simulink model "gm_sampleModel1959_2_sub"  (R2023a)
settings: Solver=VariableStepAuto  StartTime=0.0  StopTime=10.0  RelTol=1e-3
libraries: simulink x1
settings Model: Creator=user1  LastModifiedBy=user1
settings OptimizationCC: BlockReduction=off  ConditionallyExecuteInputs=off
settings DebuggingCC: InheritedTsInSrcMsg=none

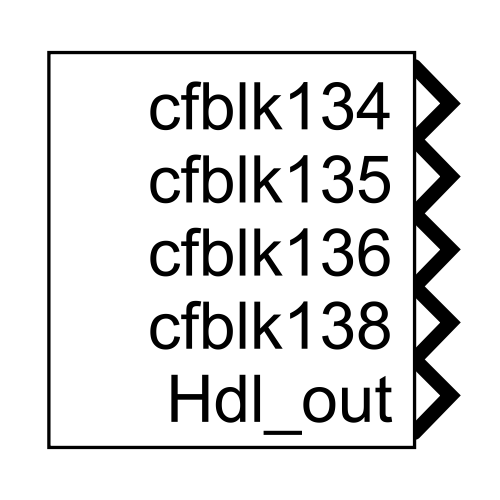
[thumbnail: Simulink's stored preview of the top-level diagram]
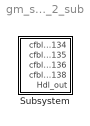
== system gm_sampleModel1959_2_sub ==
  Subsystem : Subsystem

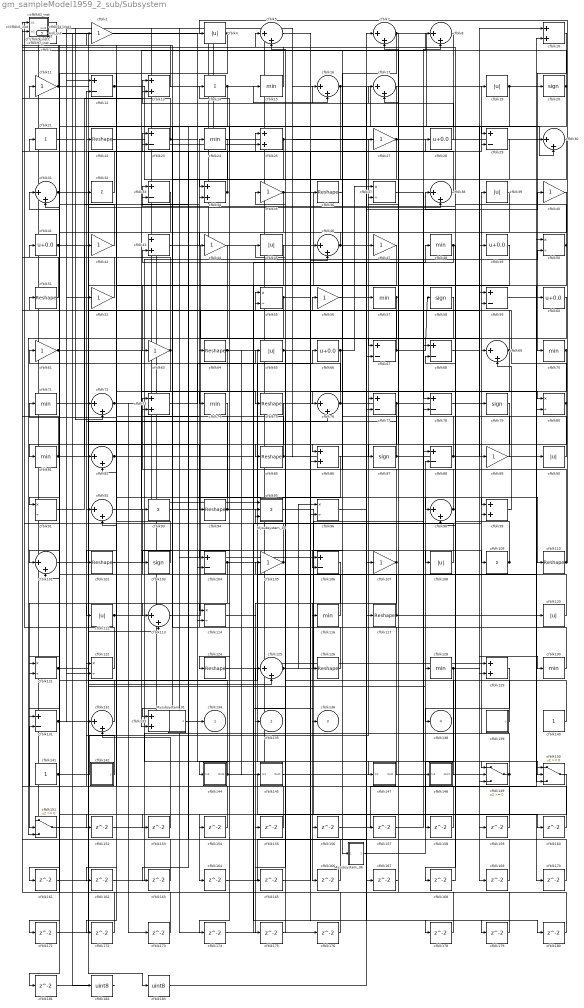
== system gm_sampleModel1959_2_sub/Subsystem ==
  Mysubsystem_15 : Subsystem
  Mysubsystem_31 : Subsystem
  Mysubsystem_36 : Subsystem
  cfblk1 : simulink/Logic and Bit Operations/Bit Clear  iBit=0
      settings: LibrarySourceBlock=|
      | hdlsllib/Logic and Bit
      | Operations/Bit Clear
  cfblk{10,13,25,34,43,73,86,99,129,133} (10 alike) : Sum  OutDataTypeStr=uint8
  cfblk100_inst : Subsystem
  cfblk{5,7..8,16..17,30..31,38,46,69,72,76,82,92,98,101,113,125,132} (19 alike) : Sum  Inputs=|++  OutDataTypeStr=uint8
  cfblk{22,36,51,64,75,85,94,102,110,117,124,126} (12 alike) : Reshape
  cfblk{20,58,79,87,103} (5 alike) : Signum
  cfblk{12,23,29,33,59,67..68,77..78,88,104,106,131} (13 alike) : Sum  Inputs=+-  OutDataTypeStr=uint8
  cfblk{2,11,27,35,40,42,44,47,52,56,61,63,89,105,107} (15 alike) : Gain  OutDataTypeStr=uint8
  cfblk{4,19,39,45,65,90,108,112,120} (9 alike) : Abs  OutDataTypeStr=uint8  SaturateOnIntegerOverflow=off
  cfblk{14,21,32,93,95,109} (6 alike) : Sum  Inputs=+  OutDataTypeStr=uint8
  cfblk111_inst : Subsystem
  cfblk{37,50,55,80,91,96,114,121..122} (9 alike) : Product  Inputs=*/  OutDataTypeStr=uint8  RndMeth=Zero  SaturateOnIntegerOverflow=on
  cfblk115_inst : Subsystem
  cfblk{15,24,48,57,70..71,74,81,116,128,130} (11 alike) : MinMax  OutDataTypeStr=uint8
  cfblk119_inst : Subsystem
  cfblk127_inst : Subsystem
  cfblk139 : Subsystem  mask(Counter Free-Running){NumBits=double(16), tsamp=double(-1)}
      mask prompts: NumBits "Simulink:masks:NumberOfBits_MP"; tsamp "Simulink:masks:SampleTime_MP"
      mask help: Simulink:masks:CounterFreeRunning_MD
  cfblk140 : Constant  OutDataTypeStr=uint8  SampleTime=-1
  cfblk141 : Constant  OutDataTypeStr=uint8  SampleTime=-1
  cfblk142 : Subsystem  mask(Counter Limited){uplimit=double(7), tsamp=double(-1)}
      mask prompts: uplimit "Simulink:masks:UpperLimit_MP"; tsamp "Simulink:masks:SampleTime_MP"
      mask help: Simulink:masks:CounterLimited_MD
      mask init:
      | nbits = double(8);
      | tsamp = double(-1);
      | uplimit = double(7);
  cfblk144 : Subsystem
  cfblk145 : Subsystem
  cfblk147 : Subsystem
  cfblk148 : Subsystem
  cfblk149 : Switch  OutDataTypeStr=uint8  SaturateOnIntegerOverflow=off  InputSameDT=off
  cfblk150 : Switch  OutDataTypeStr=uint8  SaturateOnIntegerOverflow=off  InputSameDT=off
  cfblk151 : Switch  OutDataTypeStr=uint8  SaturateOnIntegerOverflow=off  InputSameDT=off
  cfblk{152..176,178..181} (29 alike) : Delay  SampleTime=1
  cfblk182 : DataTypeConversion  OutDataTypeStr=uint8  SaturateOnIntegerOverflow=off  RndMeth=Floor
  cfblk183 : DataTypeConversion  OutDataTypeStr=uint8  SaturateOnIntegerOverflow=off  RndMeth=Floor
  cfblk18_inst : Subsystem
  cfblk26_inst : Subsystem
  cfblk{28,41,49,60,66} (5 alike) : Bias  Bias=0.0  SaturateOnIntegerOverflow=off
  cfblk3_inst : Subsystem
  cfblk53_inst : Subsystem
  cfblk54_inst : Subsystem
  cfblk62_inst : Subsystem
  cfblk6_inst : Subsystem
  cfblk97_inst : Subsystem
  cfblk9_inst : Subsystem
  cfblk134 : Outport  OutDataTypeStr=uint8  SampleTime=1  VectorParamsAs1DForOutWhenUnconnected=off
  cfblk135 : Outport  Port=2  OutDataTypeStr=uint8  SampleTime=1  VectorParamsAs1DForOutWhenUnconnected=off
  cfblk136 : Outport  Port=3  OutDataTypeStr=uint8  SampleTime=1  VectorParamsAs1DForOutWhenUnconnected=off
  cfblk138 : Outport  Port=4  OutDataTypeStr=uint8  SampleTime=1  VectorParamsAs1DForOutWhenUnconnected=off
  Hdl_out : Outport  Port=5  OutDataTypeStr=uint8  SampleTime=1
  wires:
  Mysubsystem_15/1(Out1) -> cfblk160/1
  Mysubsystem_31/1(cfblk134) -> cfblk134/1
  Mysubsystem_36/1(Out1) -> cfblk88/2
  cfblk1/1 -> cfblk183/1
  cfblk10/1 -> cfblk70/1
  cfblk100_inst/1(out1) -> cfblk12/1
  cfblk101/1 -> cfblk125/2
  cfblk102/1 -> cfblk50/2
  cfblk103/1 -> cfblk71/1
  cfblk104/1 -> cfblk151/2, cfblk149/1
  cfblk105/1 -> cfblk66/1, cfblk53_inst/1(in1)
  cfblk106/1 -> cfblk175/1
  cfblk107/1 -> cfblk73/1, cfblk166/1, Mysubsystem_15/2(In2)
  cfblk108/1 -> Mysubsystem_15/3(In3)
  cfblk109/1 -> cfblk33/1, cfblk100_inst/1(in1)
  cfblk11/1 -> cfblk62_inst/1(in1), cfblk38/2
  cfblk110/1 -> cfblk4/1, cfblk17/2
  cfblk111_inst/1(out1) -> cfblk15/1
  cfblk112/1 -> cfblk147/1(In1), cfblk24/1
  cfblk113/1 -> cfblk56/1
  cfblk114/1 -> cfblk155/1
  cfblk115_inst/1(out1) -> cfblk9_inst/1(in1), cfblk72/2, cfblk149/2
  cfblk116/1 -> cfblk12/2
  cfblk117/1 -> cfblk120/1, cfblk61/1
  cfblk119_inst/1(out1) -> cfblk176/1
  cfblk12/1 -> cfblk86/2, cfblk96/2
  cfblk120/1 -> cfblk93/1
  cfblk121/1 -> cfblk76/2, cfblk55/1
  cfblk122/1 -> cfblk18_inst/2(in2)
  cfblk124/1 -> cfblk27/1
  cfblk125/1 -> cfblk88/1, cfblk96/1
  cfblk126/1 -> cfblk2/1
  cfblk127_inst/1(out1) -> cfblk47/1
  cfblk128/1 -> cfblk159/1, cfblk158/1
  cfblk129/1 -> cfblk138/1
  cfblk13/1 -> cfblk115_inst/1(in1)
  cfblk130/1 -> cfblk45/1
  cfblk131/1 -> cfblk73/2, cfblk113/2, cfblk128/1
  cfblk132/1 -> cfblk31/2
  cfblk133/1 -> cfblk43/1
  cfblk139/1(y) -> cfblk25/1
  cfblk14/1 -> cfblk16/2, cfblk133/1
  cfblk140/1 -> cfblk38/1
  cfblk141/1 -> cfblk77/1, cfblk101/2
  cfblk142/1(y) -> cfblk22/1
  cfblk144/1(Out1) -> cfblk41/1, cfblk170/1
  cfblk145/1(Out1) -> cfblk179/1
  cfblk147/1(Out1) -> cfblk64/1
  cfblk148/1(Out1) -> cfblk105/1
  cfblk149/1 -> cfblk39/1, cfblk161/1
  cfblk15/1 -> cfblk5/1
  cfblk150/1 -> cfblk164/1
  cfblk151/1 -> cfblk19/1
  cfblk152/1 -> cfblk69/1
  cfblk153/1 -> cfblk132/2
  cfblk154/1 -> cfblk122/1
  cfblk155/1 -> cfblk6_inst/2(in2)
  cfblk156/1 -> cfblk50/1
  cfblk157/1 -> cfblk78/2
  cfblk158/1 -> cfblk92/1
  cfblk159/1 -> cfblk33/2
  cfblk16/1 -> cfblk149/3, cfblk113/1, cfblk167/1
  cfblk160/1 -> cfblk131/2
  cfblk161/1 -> cfblk10/2
  cfblk162/1 -> cfblk8/2
  cfblk163/1 -> cfblk54_inst/2(in2)
  cfblk164/1 -> cfblk67/2
  cfblk165/1 -> cfblk46/2
  cfblk166/1 -> cfblk23/1
  cfblk167/1 -> cfblk37/2
  cfblk168/1 -> cfblk68/2
  cfblk169/1 -> cfblk26_inst/2(in2)
  cfblk17/1 -> cfblk154/1
  cfblk170/1 -> cfblk5/2
  cfblk171/1 -> cfblk125/1
  cfblk172/1 -> cfblk18_inst/1(in1)
  cfblk173/1 -> cfblk111_inst/2(in2)
  cfblk174/1 -> cfblk99/2
  cfblk175/1 -> cfblk55/2
  cfblk176/1 -> cfblk31/1
  cfblk178/1 -> cfblk7/2
  cfblk179/1 -> cfblk97_inst/2(in2)
  cfblk18_inst/1(out1) -> cfblk25/2
  cfblk180/1 -> cfblk3_inst/1(in1)
  cfblk181/1 -> cfblk182/1
  cfblk182/1 -> cfblk1/1
  cfblk183/1 -> cfblk7/1
  cfblk19/1 -> cfblk163/1, cfblk162/1
  cfblk2/1 -> cfblk99/1
  cfblk20/1 -> cfblk62_inst/2(in2), cfblk156/1
  cfblk21/1 -> cfblk29/1
  cfblk22/1 -> cfblk57/1
  cfblk23/1 -> cfblk115_inst/2(in2), cfblk148/1(In1)
  cfblk24/1 -> cfblk103/1
  cfblk25/1 -> cfblk23/2, cfblk153/1
  cfblk26_inst/1(out1) -> cfblk52/1
  cfblk27/1 -> cfblk174/1, Hdl_out/1
  cfblk28/1 -> cfblk13/1
  cfblk29/1 -> cfblk144/1(In1)
  cfblk3_inst/1(out1) -> cfblk90/1, Mysubsystem_15/1(In1)
  cfblk30/1 -> cfblk34/1
  cfblk31/1 -> cfblk63/1, cfblk32/1
  cfblk32/1 -> cfblk26_inst/1(in1)
  cfblk33/1 -> cfblk131/1
  cfblk34/1 -> cfblk119_inst/2(in2), cfblk119_inst/1(in1)
  cfblk35/1 -> cfblk80/2, cfblk121/2, cfblk81/1
  cfblk36/1 -> cfblk116/1
  cfblk37/1 -> cfblk78/1
  cfblk38/1 -> cfblk14/1
  cfblk39/1 -> cfblk114/1
  cfblk4/1 -> cfblk172/1, cfblk121/1
  cfblk40/1 -> cfblk77/2
  cfblk41/1 -> cfblk82/1, cfblk169/1
  cfblk42/1 -> cfblk111_inst/1(in1)
  cfblk43/1 -> cfblk89/1
  cfblk44/1 -> cfblk171/1
  cfblk45/1 -> cfblk92/2
  cfblk46/1 -> cfblk117/1, cfblk44/1
  cfblk47/1 -> cfblk95/1
  cfblk48/1 -> cfblk98/2, cfblk43/2
  cfblk49/1 -> cfblk67/1
  cfblk5/1 -> cfblk126/1
  cfblk50/1 -> cfblk60/1, cfblk53_inst/2(in2)
  cfblk51/1 -> cfblk100_inst/2(in2)
  cfblk52/1 -> cfblk42/1
  cfblk53_inst/1(out1) -> cfblk20/1, cfblk151/1
  cfblk54_inst/1(out1) -> cfblk97_inst/1(in1), cfblk79/1
  cfblk55/1 -> cfblk28/1, cfblk104/1
  cfblk56/1 -> cfblk107/1
  cfblk57/1 -> cfblk151/3, cfblk91/1
  cfblk58/1 -> cfblk74/1
  cfblk59/1 -> cfblk150/3
  cfblk6_inst/1(out1) -> cfblk132/1
  cfblk60/1 -> cfblk86/1
  cfblk61/1 -> cfblk29/2, cfblk109/1
  cfblk62_inst/1(out1) -> cfblk46/1, cfblk129/1
  cfblk63/1 -> cfblk82/2, cfblk127_inst/2(in2), cfblk127_inst/1(in1)
  cfblk64/1 -> cfblk110/1, cfblk102/1, cfblk145/1(In1)
  cfblk65/1 -> cfblk108/1, cfblk80/1, cfblk165/1
  cfblk66/1 -> cfblk133/2, cfblk106/2, cfblk37/1
  cfblk67/1 -> cfblk58/1, cfblk35/1
  cfblk68/1 -> cfblk49/1
  cfblk69/1 -> cfblk3_inst/2(in2), cfblk135/1
  cfblk7/1 -> cfblk87/1, cfblk76/1, cfblk30/2
  cfblk70/1 -> cfblk129/2, cfblk112/1
  cfblk71/1 -> cfblk94/1
  cfblk72/1 -> cfblk75/1, cfblk173/1
  cfblk73/1 -> cfblk65/1
  cfblk74/1 -> cfblk152/1
  cfblk75/1 -> cfblk124/1
  cfblk76/1 -> cfblk40/1, cfblk11/1, Mysubsystem_36/1(In1)
  cfblk77/1 -> cfblk85/1, cfblk150/2
  cfblk78/1 -> cfblk130/1
  cfblk79/1 -> cfblk181/1
  cfblk8/1 -> cfblk101/1
  cfblk80/1 -> cfblk59/2, cfblk104/2
  cfblk81/1 -> cfblk54_inst/1(in1), cfblk34/2
  cfblk82/1 -> cfblk136/1, cfblk48/1
  cfblk85/1 -> cfblk98/1, cfblk178/1, cfblk21/1
  cfblk86/1 -> cfblk114/2
  cfblk87/1 -> cfblk72/1, cfblk6_inst/1(in1)
  cfblk88/1 -> cfblk17/1, cfblk10/1
  cfblk89/1 -> cfblk51/1
  cfblk9_inst/1(out1) -> cfblk30/1, cfblk106/1
  cfblk90/1 -> cfblk68/1
  cfblk91/1 -> cfblk13/2
  cfblk92/1 -> cfblk8/1
  cfblk93/1 -> cfblk150/1
  cfblk94/1 -> cfblk9_inst/2(in2), cfblk59/1, cfblk180/1
  cfblk95/1 -> cfblk36/1
  cfblk96/1 -> cfblk157/1
  cfblk97_inst/1(out1) -> cfblk91/2, cfblk122/2
  cfblk98/1 -> cfblk16/1, cfblk168/1
  cfblk99/1 -> cfblk69/2

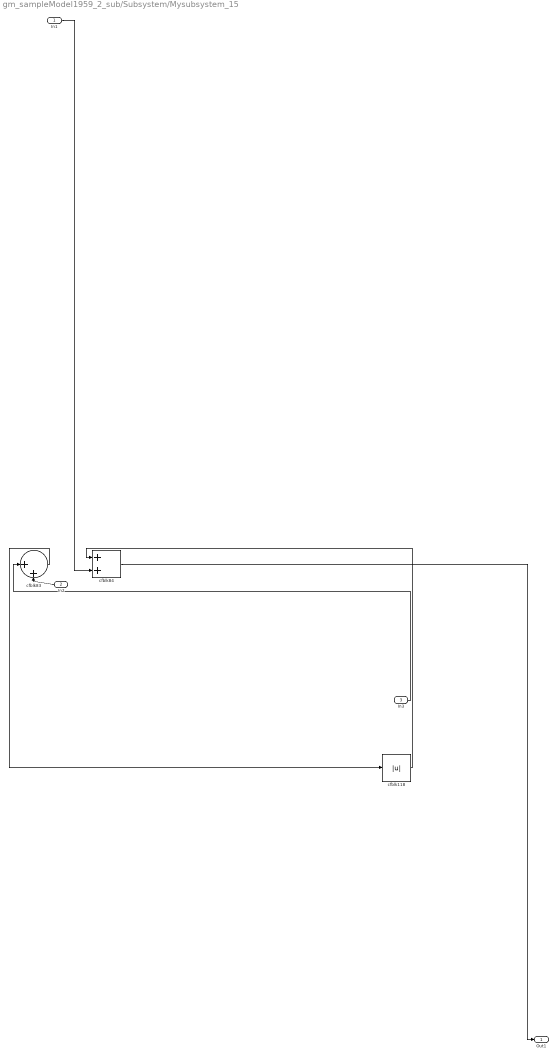
== system gm_sampleModel1959_2_sub/Subsystem/Mysubsystem_15 ==
  In1 : Inport  OutDataTypeStr=uint8  PortDimensions=1  SampleTime=1
  In2 : Inport  Port=2  OutDataTypeStr=uint8  PortDimensions=1  SampleTime=1
  In3 : Inport  Port=3  OutDataTypeStr=uint8  PortDimensions=1  SampleTime=1
  cfblk118 : Abs  SaturateOnIntegerOverflow=off
  cfblk83 : Sum  Inputs=|++
  cfblk84 : Sum
  Out1 : Outport  SampleTime=1
  wires:
  In1/1 -> cfblk84/2
  In2/1 -> cfblk83/2
  In3/1 -> cfblk83/1
  cfblk118/1 -> cfblk84/1
  cfblk83/1 -> cfblk118/1
  cfblk84/1 -> Out1/1

== system gm_sampleModel1959_2_sub/Subsystem/Mysubsystem_31 ==
  cfblk123 : Abs  SaturateOnIntegerOverflow=off
  cfblk143 : Subsystem  mask(Counter Limited){uplimit=double(7), tsamp=double(-1)}
      mask prompts: uplimit "Simulink:masks:UpperLimit_MP"; tsamp "Simulink:masks:SampleTime_MP"
      mask help: Simulink:masks:CounterLimited_MD
      mask init:
      | nbits = double(8);
      | tsamp = double(-1);
      | uplimit = double(7);
  cfblk134 : Outport  SampleTime=1  VectorParamsAs1DForOutWhenUnconnected=off
  wires:
  cfblk123/1 -> cfblk134/1
  cfblk143/1(y) -> cfblk123/1

== system gm_sampleModel1959_2_sub/Subsystem/Mysubsystem_36 ==
  In1 : Inport  OutDataTypeStr=uint8  PortDimensions=1  SampleTime=1
  cfblk146 : Subsystem
  cfblk177 : Delay  SampleTime=1
  Out1 : Outport  SampleTime=1
  wires:
  In1/1 -> cfblk146/1(In1)
  cfblk146/1(Out1) -> cfblk177/1
  cfblk177/1 -> Out1/1

== system gm_sampleModel1959_2_sub/Subsystem/cfblk100_inst ==
  in1 : Inport  OutDataTypeStr=uint8  SampleTime=1
  in2 : Inport  Port=2  OutDataTypeStr=uint8  SampleTime=1
  mul_cfblk100_dotp_mulcomp : Product  Inputs=**  OutDataTypeStr=uint8  SampleTime=1
  out1 : Outport  OutDataTypeStr=uint8  SampleTime=1
  wires:
  in1/1 -> mul_cfblk100_dotp_mulcomp/1
  in2/1 -> mul_cfblk100_dotp_mulcomp/2
  mul_cfblk100_dotp_mulcomp/1 -> out1/1

== system gm_sampleModel1959_2_sub/Subsystem/cfblk111_inst ==
  in1 : Inport  OutDataTypeStr=uint8  SampleTime=1
  in2 : Inport  Port=2  OutDataTypeStr=uint8  SampleTime=1
  mul_cfblk111_dotp_mulcomp : Product  Inputs=**  OutDataTypeStr=uint8  SampleTime=1
  out1 : Outport  OutDataTypeStr=uint8  SampleTime=1
  wires:
  in1/1 -> mul_cfblk111_dotp_mulcomp/1
  in2/1 -> mul_cfblk111_dotp_mulcomp/2
  mul_cfblk111_dotp_mulcomp/1 -> out1/1

== system gm_sampleModel1959_2_sub/Subsystem/cfblk115_inst ==
  in1 : Inport  OutDataTypeStr=uint8  SampleTime=1
  in2 : Inport  Port=2  OutDataTypeStr=uint8  SampleTime=1
  mul_cfblk115_dotp_mulcomp : Product  Inputs=**  OutDataTypeStr=uint8  SampleTime=1
  out1 : Outport  OutDataTypeStr=uint8  SampleTime=1
  wires:
  in1/1 -> mul_cfblk115_dotp_mulcomp/1
  in2/1 -> mul_cfblk115_dotp_mulcomp/2
  mul_cfblk115_dotp_mulcomp/1 -> out1/1

== system gm_sampleModel1959_2_sub/Subsystem/cfblk119_inst ==
  in1 : Inport  OutDataTypeStr=uint8  SampleTime=1
  in2 : Inport  Port=2  OutDataTypeStr=uint8  SampleTime=1
  mul_cfblk119_dotp_mulcomp : Product  Inputs=**  OutDataTypeStr=uint8  SampleTime=1
  out1 : Outport  OutDataTypeStr=uint8  SampleTime=1
  wires:
  in1/1 -> mul_cfblk119_dotp_mulcomp/1
  in2/1 -> mul_cfblk119_dotp_mulcomp/2
  mul_cfblk119_dotp_mulcomp/1 -> out1/1

== system gm_sampleModel1959_2_sub/Subsystem/cfblk127_inst ==
  in1 : Inport  OutDataTypeStr=uint8  SampleTime=1
  in2 : Inport  Port=2  OutDataTypeStr=uint8  SampleTime=1
  mul_cfblk127_dotp_mulcomp : Product  Inputs=**  OutDataTypeStr=uint8  SampleTime=1
  out1 : Outport  OutDataTypeStr=uint8  SampleTime=1
  wires:
  in1/1 -> mul_cfblk127_dotp_mulcomp/1
  in2/1 -> mul_cfblk127_dotp_mulcomp/2
  mul_cfblk127_dotp_mulcomp/1 -> out1/1

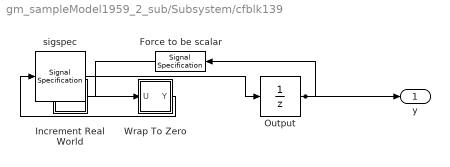
== system gm_sampleModel1959_2_sub/Subsystem/cfblk139 ==
  Force to be scalar : SignalSpecification  DisableCoverage=on  Dimensions=1
  Increment Real World : Subsystem  mask(Real World Value Increment){}
      mask help: Simulink:masks:RealWorldValueIncrement_MD
      mask Display: disp('V++')
  Output : UnitDelay  InitialCondition=0.0  SampleTime=tsamp  HasFrameUpgradeWarning=on
  Wrap To Zero : Subsystem  mask(Wrap To Zero){Threshold=double(65535)}
      mask prompts: Threshold "Simulink:masks:Threshold_MP"
      mask help: Simulink:masks:WrapToZero_MD
  sigspec : SignalSpecification  OutDataTypeStr=uint16  Dimensions=1
  y : Outport  SampleTime=1
  wires:
  Force to be scalar/1 -> Increment Real World/1(u)
  Increment Real World/1(y) -> Wrap To Zero/1(U)
  Output/1 -> Force to be scalar/1, y/1
  Wrap To Zero/1(Y) -> sigspec/1
  sigspec/1 -> Output/1

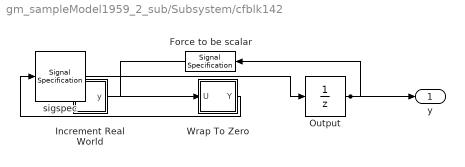
== system gm_sampleModel1959_2_sub/Subsystem/cfblk142 ==
  Force to be scalar : SignalSpecification  DisableCoverage=on  Dimensions=1
  Increment Real World : Subsystem  mask(Real World Value Increment){}
      mask help: Simulink:masks:RealWorldValueIncrement_MD
      mask Display: disp('V++')
  Output : UnitDelay  InitialCondition=0.0  SampleTime=tsamp  HasFrameUpgradeWarning=on
  Wrap To Zero : Subsystem  mask(Wrap To Zero){Threshold=double(7)}
      mask prompts: Threshold "Simulink:masks:Threshold_MP"
      mask help: Simulink:masks:WrapToZero_MD
  sigspec : SignalSpecification  OutDataTypeStr=uint8  Dimensions=1
  y : Outport  SampleTime=1
  wires:
  Force to be scalar/1 -> Increment Real World/1(u)
  Increment Real World/1(y) -> Wrap To Zero/1(U)
  Output/1 -> Force to be scalar/1, y/1
  Wrap To Zero/1(Y) -> sigspec/1
  sigspec/1 -> Output/1

== system gm_sampleModel1959_2_sub/Subsystem/cfblk144 ==
  In1 : Inport  OutDataTypeStr=uint8  PortDimensions=1  SampleTime=1
  Out1 : Outport  SampleTime=1
  wires:
  In1/1 -> Out1/1

== system gm_sampleModel1959_2_sub/Subsystem/cfblk145 ==
  In1 : Inport  OutDataTypeStr=uint8  PortDimensions=1  SampleTime=1
  Out1 : Outport  SampleTime=1
  wires:
  In1/1 -> Out1/1

== system gm_sampleModel1959_2_sub/Subsystem/cfblk147 ==
  In1 : Inport  OutDataTypeStr=uint8  PortDimensions=1  SampleTime=1
  Out1 : Outport  SampleTime=1
  wires:
  In1/1 -> Out1/1

== system gm_sampleModel1959_2_sub/Subsystem/cfblk148 ==
  In1 : Inport  OutDataTypeStr=uint8  PortDimensions=1  SampleTime=1
  Out1 : Outport  SampleTime=1
  wires:
  In1/1 -> Out1/1

== system gm_sampleModel1959_2_sub/Subsystem/cfblk18_inst ==
  in1 : Inport  OutDataTypeStr=uint8  SampleTime=1
  in2 : Inport  Port=2  OutDataTypeStr=uint8  SampleTime=1
  mul_cfblk18_dotp_mulcomp : Product  Inputs=**  OutDataTypeStr=uint8  SampleTime=1
  out1 : Outport  OutDataTypeStr=uint8  SampleTime=1
  wires:
  in1/1 -> mul_cfblk18_dotp_mulcomp/1
  in2/1 -> mul_cfblk18_dotp_mulcomp/2
  mul_cfblk18_dotp_mulcomp/1 -> out1/1

== system gm_sampleModel1959_2_sub/Subsystem/cfblk26_inst ==
  in1 : Inport  OutDataTypeStr=uint8  SampleTime=1
  in2 : Inport  Port=2  OutDataTypeStr=uint8  SampleTime=1
  mul_cfblk26_dotp_mulcomp : Product  Inputs=**  OutDataTypeStr=uint8  SampleTime=1
  out1 : Outport  OutDataTypeStr=uint8  SampleTime=1
  wires:
  in1/1 -> mul_cfblk26_dotp_mulcomp/1
  in2/1 -> mul_cfblk26_dotp_mulcomp/2
  mul_cfblk26_dotp_mulcomp/1 -> out1/1

== system gm_sampleModel1959_2_sub/Subsystem/cfblk3_inst ==
  in1 : Inport  OutDataTypeStr=uint8  SampleTime=1
  in2 : Inport  Port=2  OutDataTypeStr=uint8  SampleTime=1
  mul_cfblk3_dotp_mulcomp : Product  Inputs=**  OutDataTypeStr=uint8  SampleTime=1
  out1 : Outport  OutDataTypeStr=uint8  SampleTime=1
  wires:
  in1/1 -> mul_cfblk3_dotp_mulcomp/1
  in2/1 -> mul_cfblk3_dotp_mulcomp/2
  mul_cfblk3_dotp_mulcomp/1 -> out1/1

== system gm_sampleModel1959_2_sub/Subsystem/cfblk53_inst ==
  in1 : Inport  OutDataTypeStr=uint8  SampleTime=1
  in2 : Inport  Port=2  OutDataTypeStr=uint8  SampleTime=1
  mul_cfblk53_dotp_mulcomp : Product  Inputs=**  OutDataTypeStr=uint8  SampleTime=1
  out1 : Outport  OutDataTypeStr=uint8  SampleTime=1
  wires:
  in1/1 -> mul_cfblk53_dotp_mulcomp/1
  in2/1 -> mul_cfblk53_dotp_mulcomp/2
  mul_cfblk53_dotp_mulcomp/1 -> out1/1

== system gm_sampleModel1959_2_sub/Subsystem/cfblk54_inst ==
  in1 : Inport  OutDataTypeStr=uint8  SampleTime=1
  in2 : Inport  Port=2  OutDataTypeStr=uint8  SampleTime=1
  mul_cfblk54_dotp_mulcomp : Product  Inputs=**  OutDataTypeStr=uint8  SampleTime=1
  out1 : Outport  OutDataTypeStr=uint8  SampleTime=1
  wires:
  in1/1 -> mul_cfblk54_dotp_mulcomp/1
  in2/1 -> mul_cfblk54_dotp_mulcomp/2
  mul_cfblk54_dotp_mulcomp/1 -> out1/1

== system gm_sampleModel1959_2_sub/Subsystem/cfblk62_inst ==
  in1 : Inport  OutDataTypeStr=uint8  SampleTime=1
  in2 : Inport  Port=2  OutDataTypeStr=uint8  SampleTime=1
  mul_cfblk62_dotp_mulcomp : Product  Inputs=**  OutDataTypeStr=uint8  SampleTime=1
  out1 : Outport  OutDataTypeStr=uint8  SampleTime=1
  wires:
  in1/1 -> mul_cfblk62_dotp_mulcomp/1
  in2/1 -> mul_cfblk62_dotp_mulcomp/2
  mul_cfblk62_dotp_mulcomp/1 -> out1/1

== system gm_sampleModel1959_2_sub/Subsystem/cfblk6_inst ==
  in1 : Inport  OutDataTypeStr=uint8  SampleTime=1
  in2 : Inport  Port=2  OutDataTypeStr=uint8  SampleTime=1
  mul_cfblk6_dotp_mulcomp : Product  Inputs=**  OutDataTypeStr=uint8  SampleTime=1
  out1 : Outport  OutDataTypeStr=uint8  SampleTime=1
  wires:
  in1/1 -> mul_cfblk6_dotp_mulcomp/1
  in2/1 -> mul_cfblk6_dotp_mulcomp/2
  mul_cfblk6_dotp_mulcomp/1 -> out1/1

== system gm_sampleModel1959_2_sub/Subsystem/cfblk97_inst ==
  in1 : Inport  OutDataTypeStr=uint8  SampleTime=1
  in2 : Inport  Port=2  OutDataTypeStr=uint8  SampleTime=1
  mul_cfblk97_dotp_mulcomp : Product  Inputs=**  OutDataTypeStr=uint8  SampleTime=1
  out1 : Outport  OutDataTypeStr=uint8  SampleTime=1
  wires:
  in1/1 -> mul_cfblk97_dotp_mulcomp/1
  in2/1 -> mul_cfblk97_dotp_mulcomp/2
  mul_cfblk97_dotp_mulcomp/1 -> out1/1

== system gm_sampleModel1959_2_sub/Subsystem/cfblk9_inst ==
  in1 : Inport  OutDataTypeStr=uint8  SampleTime=1
  in2 : Inport  Port=2  OutDataTypeStr=uint8  SampleTime=1
  mul_cfblk9_dotp_mulcomp : Product  Inputs=**  OutDataTypeStr=uint8  SampleTime=1
  out1 : Outport  OutDataTypeStr=uint8  SampleTime=1
  wires:
  in1/1 -> mul_cfblk9_dotp_mulcomp/1
  in2/1 -> mul_cfblk9_dotp_mulcomp/2
  mul_cfblk9_dotp_mulcomp/1 -> out1/1

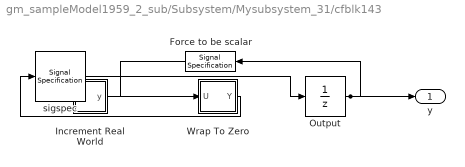
== system gm_sampleModel1959_2_sub/Subsystem/Mysubsystem_31/cfblk143 ==
  Force to be scalar : SignalSpecification  DisableCoverage=on  Dimensions=1
  Increment Real World : Subsystem  mask(Real World Value Increment){}
      mask help: Simulink:masks:RealWorldValueIncrement_MD
      mask Display: disp('V++')
  Output : UnitDelay  InitialCondition=0.0  SampleTime=tsamp  HasFrameUpgradeWarning=on
  Wrap To Zero : Subsystem  mask(Wrap To Zero){Threshold=double(7)}
      mask prompts: Threshold "Simulink:masks:Threshold_MP"
      mask help: Simulink:masks:WrapToZero_MD
  sigspec : SignalSpecification  OutDataTypeStr=uint8  Dimensions=1
  y : Outport  SampleTime=1
  wires:
  Force to be scalar/1 -> Increment Real World/1(u)
  Increment Real World/1(y) -> Wrap To Zero/1(U)
  Output/1 -> Force to be scalar/1, y/1
  Wrap To Zero/1(Y) -> sigspec/1
  sigspec/1 -> Output/1

== system gm_sampleModel1959_2_sub/Subsystem/Mysubsystem_36/cfblk146 ==
  In1 : Inport  OutDataTypeStr=uint8  PortDimensions=1  SampleTime=1
  Out1 : Outport  SampleTime=1
  wires:
  In1/1 -> Out1/1

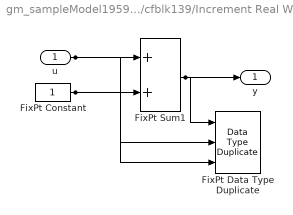
== system gm_sampleModel1959_2_sub/Subsystem/cfblk139/Increment Real World ==
  u : Inport  OutDataTypeStr=uint16  SampleTime=1
  FixPt Constant : Constant  DisableCoverage=on  OutDataTypeStr=Inherit: Inherit via back propagation  SampleTime=-1
  FixPt Data Type Duplicate : DataTypeDuplicate  DisableCoverage=on  NumInputPorts=3
  FixPt Sum1 : Sum  InputSameDT=on  OutDataTypeStr=Inherit: Inherit via back propagation  LockScale=on
  y : Outport  SampleTime=1
  wires:
  u/1 -> FixPt Sum1/1, FixPt Data Type Duplicate/2
  FixPt Constant/1 -> FixPt Sum1/2, FixPt Data Type Duplicate/3
  FixPt Sum1/1 -> FixPt Data Type Duplicate/1, y/1

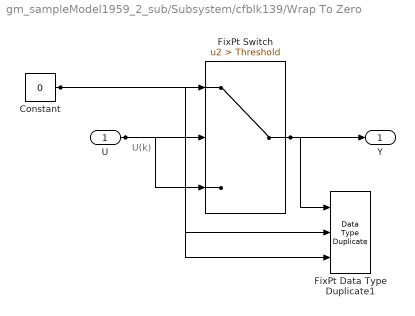
== system gm_sampleModel1959_2_sub/Subsystem/cfblk139/Wrap To Zero ==
  note: U(k)
  U : Inport  OutDataTypeStr=uint16  SampleTime=1
  Constant : Constant  DisableCoverage=on  Value=0  OutDataTypeStr=Inherit: Inherit via back propagation  SampleTime=-1
  FixPt Data Type Duplicate1 : DataTypeDuplicate  DisableCoverage=on  NumInputPorts=3
  FixPt Switch : Switch  Criteria=u2 > Threshold  Threshold=Threshold  OutDataTypeStr=Inherit: Inherit via back propagation  ZeroCross=off  SaturateOnIntegerOverflow=off  InputSameDT=off
  Y : Outport  SampleTime=1
  wires:
  U/1 -> FixPt Switch/3, FixPt Switch/2, FixPt Data Type Duplicate1/2
  Constant/1 -> FixPt Switch/1, FixPt Data Type Duplicate1/3
  FixPt Switch/1 -> FixPt Data Type Duplicate1/1, Y/1

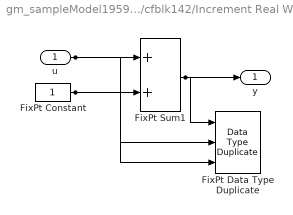
== system gm_sampleModel1959_2_sub/Subsystem/cfblk142/Increment Real World ==
  u : Inport  OutDataTypeStr=uint8  SampleTime=1
  FixPt Constant : Constant  DisableCoverage=on  OutDataTypeStr=Inherit: Inherit via back propagation  SampleTime=-1
  FixPt Data Type Duplicate : DataTypeDuplicate  DisableCoverage=on  NumInputPorts=3
  FixPt Sum1 : Sum  InputSameDT=on  OutDataTypeStr=Inherit: Inherit via back propagation  LockScale=on
  y : Outport  SampleTime=1
  wires:
  u/1 -> FixPt Sum1/1, FixPt Data Type Duplicate/2
  FixPt Constant/1 -> FixPt Sum1/2, FixPt Data Type Duplicate/3
  FixPt Sum1/1 -> FixPt Data Type Duplicate/1, y/1

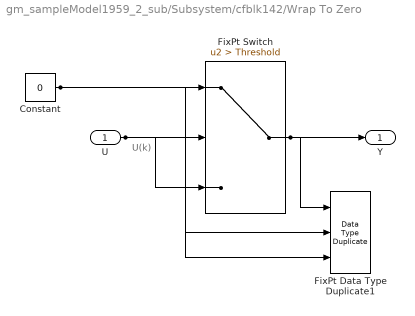
== system gm_sampleModel1959_2_sub/Subsystem/cfblk142/Wrap To Zero ==
  note: U(k)
  U : Inport  OutDataTypeStr=uint8  SampleTime=1
  Constant : Constant  DisableCoverage=on  Value=0  OutDataTypeStr=Inherit: Inherit via back propagation  SampleTime=-1
  FixPt Data Type Duplicate1 : DataTypeDuplicate  DisableCoverage=on  NumInputPorts=3
  FixPt Switch : Switch  Criteria=u2 > Threshold  Threshold=Threshold  OutDataTypeStr=Inherit: Inherit via back propagation  ZeroCross=off  SaturateOnIntegerOverflow=off  InputSameDT=off
  Y : Outport  SampleTime=1
  wires:
  U/1 -> FixPt Switch/3, FixPt Switch/2, FixPt Data Type Duplicate1/2
  Constant/1 -> FixPt Switch/1, FixPt Data Type Duplicate1/3
  FixPt Switch/1 -> FixPt Data Type Duplicate1/1, Y/1

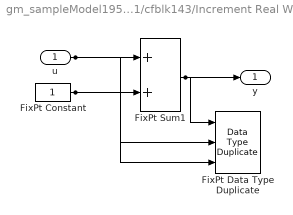
== system gm_sampleModel1959_2_sub/Subsystem/Mysubsystem_31/cfblk143/Increment Real World ==
  u : Inport  OutDataTypeStr=uint8  SampleTime=1
  FixPt Constant : Constant  DisableCoverage=on  OutDataTypeStr=Inherit: Inherit via back propagation  SampleTime=-1
  FixPt Data Type Duplicate : DataTypeDuplicate  DisableCoverage=on  NumInputPorts=3
  FixPt Sum1 : Sum  InputSameDT=on  OutDataTypeStr=Inherit: Inherit via back propagation  LockScale=on
  y : Outport  SampleTime=1
  wires:
  u/1 -> FixPt Sum1/1, FixPt Data Type Duplicate/2
  FixPt Constant/1 -> FixPt Sum1/2, FixPt Data Type Duplicate/3
  FixPt Sum1/1 -> FixPt Data Type Duplicate/1, y/1

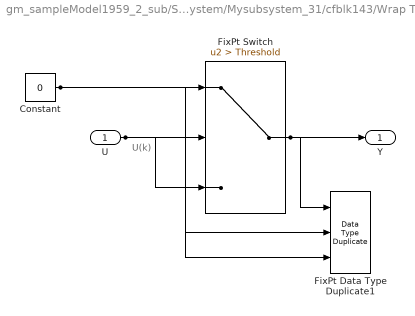
== system gm_sampleModel1959_2_sub/Subsystem/Mysubsystem_31/cfblk143/Wrap To Zero ==
  note: U(k)
  U : Inport  OutDataTypeStr=uint8  SampleTime=1
  Constant : Constant  DisableCoverage=on  Value=0  OutDataTypeStr=Inherit: Inherit via back propagation  SampleTime=-1
  FixPt Data Type Duplicate1 : DataTypeDuplicate  DisableCoverage=on  NumInputPorts=3
  FixPt Switch : Switch  Criteria=u2 > Threshold  Threshold=Threshold  OutDataTypeStr=Inherit: Inherit via back propagation  ZeroCross=off  SaturateOnIntegerOverflow=off  InputSameDT=off
  Y : Outport  SampleTime=1
  wires:
  U/1 -> FixPt Switch/3, FixPt Switch/2, FixPt Data Type Duplicate1/2
  Constant/1 -> FixPt Switch/1, FixPt Data Type Duplicate1/3
  FixPt Switch/1 -> FixPt Data Type Duplicate1/1, Y/1
